simulink model "AcasXuClosedLoop_6"  (R2019b)
settings: Solver=VariableStepAuto  StartTime=0.0  StopTime=30  RelTol=1e-3
libraries: neural x624, simulink x2
(part 1 of 33)
settings Model: Creator=manzand  LastModifiedBy=manzand

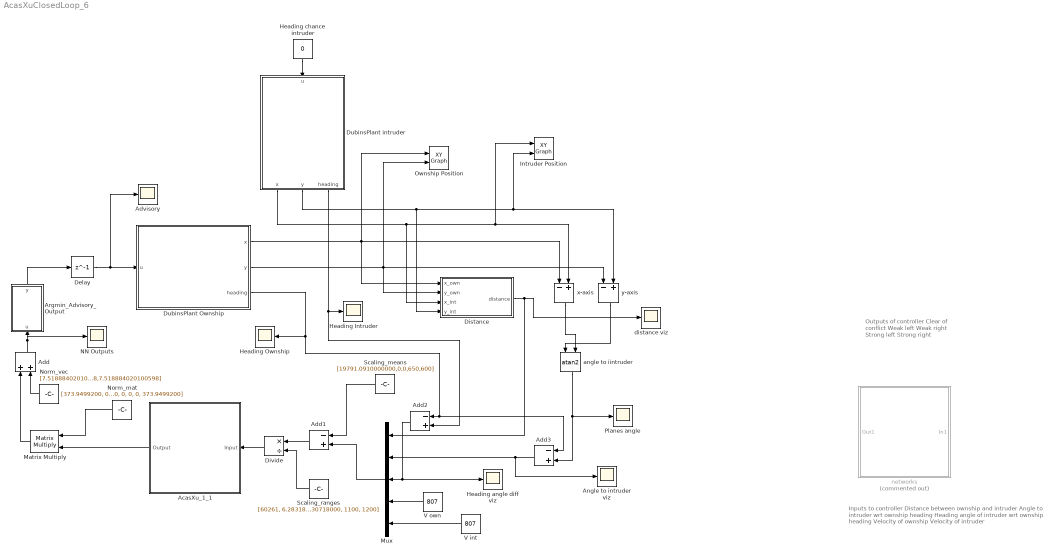
== system AcasXuClosedLoop_6 ==
  note: Outputs of controller
      | Clear of conflict
      | Weak left
      | Weak right
      | Strong left
      | Strong right
  note: Inputs to controller
      | Distance between ownship and intruder
      | Angle to intruder wrt ownship heading
      | Heading angle of intruder wrt ownship heading
      | Velocity of ownship
      | Velocity of intruder
  AcasXu_1_1 : Subsystem
      mask help: Feed-Forward Neural Network
      mask Display: e = 0.06;c1 = [120 150 230]/255;c2 = ([120 150 230]+0)/383;c3 = ([120 150 230]+128)/383;patch([0 1 1 0],[0 0 1 1],c1);patch([0 1 1 1-e 1-e 0+e],[0 0 1 1-e 0+e 0+e],c2);patch([0 0 1 1-e 0+e 0+e],[0 1 1 1-e 1-e 0+e],c3);plot([0 1 1 0 0],[0 0 1 1 0]);fprintf('NNET');port_label('input',1,' Input');port_label('output',1,'Output ');
  Add : Sum  Priority=20
  Add1 : Sum  Priority=14  Inputs=-+
  Add2 : Sum  Priority=9  Inputs=-+
  Add3 : Sum  Priority=9  Inputs=-+
  Advisory : Scope
  Angle to intruder viz : Scope
  Argmin_Advisory_Output : MATLAB Function  Priority=21  TreatAsAtomicUnit=on
  Delay : Delay  Priority=1  DelayLength=1  InitialCondition=0
  Distance : MATLAB Function  Priority=5  TreatAsAtomicUnit=on
  Divide : Product  Priority=16  Inputs=*/
  DubinsPlant Ownship : Stateflow chart  Priority=2  BlockKeywords=__PRM__SERIALIZED__DATA__:Stateflow Chart,Stateflow Diagram  TreatAsAtomicUnit=on
  DubinsPlant intruder : Stateflow chart  Priority=4  BlockKeywords=__PRM__SERIALIZED__DATA__:Stateflow Chart,Stateflow Diagram  TreatAsAtomicUnit=on
  Heading Intruder : Scope
  Heading Ownship : Scope
  Heading angle diff viz : Scope
  "Heading chance intruder " : Constant  Priority=3  Value=0
  Intruder Position : simulink/Sinks/XY Graph  xmin=0  xmax=40200  ymin=-100  ymax=100  st=-1
  Matrix Multiply : Product  Priority=19  Multiplication=Matrix(*)
  Mux : Mux  Priority=12  Inputs=5
  NN Outputs : Scope
  Norm_mat : Constant  Priority=18  Value=|  VectorParams1D=off
      | [373.9499200, 0, 0, 0, 0; 0, 373.9499200, 0, 0, 0;
      | 0, 0, 373.9499200, 0, 0;
      | 0, 0, 0, 373.9499200, 0;
      | 0, 0, 0, 0, 373.9499200]
  "Norm_vec " : Constant  Value=[7.518884020100598, 7.518884020100598,7.518884020100598,7.518884020100598,7.518884020100598]
  Ownship Position : simulink/Sinks/XY Graph  xmin=-500  xmax=8000  ymin=-100  ymax=25000  st=-1
  Planes angle : Scope
  Scaling_means : Constant  Priority=13  Value=[19791.0910000000,0,0,650,600]
  Scaling_ranges : Constant  Priority=15  Value=[60261, 6.28318530718000, 6.28318530718000, 1100, 1200]  VectorParams1D=off
  V int : Constant  Priority=11  Value=807
  V own : Constant  Priority=10  Value=807
  angle to iintruder : Trigonometry  Priority=8  Operator=atan2  OutputSignalType=real
  distance viz : Scope
  networks : Subsystem  Commented=on
  x-axis : Sum  Priority=6  Inputs=-+
  y-axis : Sum  Priority=7  Inputs=-+
  wires:
  Add2/1 -> Mux/3, Heading angle diff viz/1
  V int/1 -> Mux/5
  Mux/1 -> Add1/2
  Argmin_Advisory_Output/1(y) -> Delay/1
  angle to iintruder/1 -> Planes angle/1, Add3/2
  Distance/1(distance) -> Mux/1, distance viz/1
  Scaling_ranges/1 -> Divide/2
  Add1/1 -> Divide/1
  Matrix Multiply/1 -> Add/1
  DubinsPlant intruder/3(heading) -> Heading Intruder/1, Add2/2
  DubinsPlant Ownship/1(x) -> Distance/1(x_own), x-axis/1, Ownship Position/1
  Scaling_means/1 -> Add1/1
  DubinsPlant intruder/2(y) -> Distance/4(y_int), y-axis/2, Intruder Position/2
  "Norm_vec "/1 -> Add/2
  DubinsPlant intruder/1(x) -> Distance/3(x_int), x-axis/2, Intruder Position/1
  Delay/1 -> DubinsPlant Ownship/1(u), Advisory/1
  DubinsPlant Ownship/3(heading) -> Heading Ownship/1, Add3/1, Add2/1
  V own/1 -> Mux/4
  AcasXu_1_1/1(Output) -> Matrix Multiply/2
  "Heading chance intruder "/1 -> DubinsPlant intruder/1(u)
  DubinsPlant Ownship/2(y) -> Distance/2(y_own), y-axis/1, Ownship Position/2
  Add/1 -> NN Outputs/1, Argmin_Advisory_Output/1(u)
  Norm_mat/1 -> Matrix Multiply/1
  Divide/1 -> AcasXu_1_1/1(Input)
  Add3/1 -> Angle to intruder viz/1, Mux/2
  x-axis/1 -> angle to iintruder/2
  y-axis/1 -> angle to iintruder/1

== system AcasXuClosedLoop_6/AcasXu_1_1 ==
  Input : Inport  PortDimensions=5
      mask Display: e = 0.06;c1 = [120 230 180]/255;c2 = ([120 230 180]+0)/(256+128);c3 = ([120 230 180]+128)/(256+128);patch([0 1 1 0],[0 0 1 1],c1);patch([0 1 1 1-e 1-e 0+e],[0 0 1 1-e 0+e 0+e],c2);patch([0 0 1 1-e 0+e 0+e],[0 1 1 1-e 1-e 0+e],c3);plot([0 1 1 0 0],[0 0 1 1 0]);
  Layer 1 : Subsystem
      mask Display: e = 0.06;c1 = [120 150 230]/255;c2 = ([120 150 230]+0)/383;c3 = ([120 150 230]+128)/383;patch([0 1 1 0],[0 0 1 1],c1);patch([0 1 1 1-e 1-e 0+e],[0 0 1 1-e 0+e 0+e],c2);patch([0 0 1 1-e 0+e 0+e],[0 1 1 1-e 1-e 0+e],c3);plot([0 1 1 0 0],[0 0 1 1 0]);
  Layer 2 : Subsystem
      mask Display: e = 0.06;c1 = [120 150 230]/255;c2 = ([120 150 230]+0)/383;c3 = ([120 150 230]+128)/383;patch([0 1 1 0],[0 0 1 1],c1);patch([0 1 1 1-e 1-e 0+e],[0 0 1 1-e 0+e 0+e],c2);patch([0 0 1 1-e 0+e 0+e],[0 1 1 1-e 1-e 0+e],c3);plot([0 1 1 0 0],[0 0 1 1 0]);
  Layer 3 : Subsystem
      mask Display: e = 0.06;c1 = [120 150 230]/255;c2 = ([120 150 230]+0)/383;c3 = ([120 150 230]+128)/383;patch([0 1 1 0],[0 0 1 1],c1);patch([0 1 1 1-e 1-e 0+e],[0 0 1 1-e 0+e 0+e],c2);patch([0 0 1 1-e 0+e 0+e],[0 1 1 1-e 1-e 0+e],c3);plot([0 1 1 0 0],[0 0 1 1 0]);
  Layer 4 : Subsystem
      mask Display: e = 0.06;c1 = [120 150 230]/255;c2 = ([120 150 230]+0)/383;c3 = ([120 150 230]+128)/383;patch([0 1 1 0],[0 0 1 1],c1);patch([0 1 1 1-e 1-e 0+e],[0 0 1 1-e 0+e 0+e],c2);patch([0 0 1 1-e 0+e 0+e],[0 1 1 1-e 1-e 0+e],c3);plot([0 1 1 0 0],[0 0 1 1 0]);
  Layer 5 : Subsystem
      mask Display: e = 0.06;c1 = [120 150 230]/255;c2 = ([120 150 230]+0)/383;c3 = ([120 150 230]+128)/383;patch([0 1 1 0],[0 0 1 1],c1);patch([0 1 1 1-e 1-e 0+e],[0 0 1 1-e 0+e 0+e],c2);patch([0 0 1 1-e 0+e 0+e],[0 1 1 1-e 1-e 0+e],c3);plot([0 1 1 0 0],[0 0 1 1 0]);
  Layer 6 : Subsystem
      mask Display: e = 0.06;c1 = [120 150 230]/255;c2 = ([120 150 230]+0)/383;c3 = ([120 150 230]+128)/383;patch([0 1 1 0],[0 0 1 1],c1);patch([0 1 1 1-e 1-e 0+e],[0 0 1 1-e 0+e 0+e],c2);patch([0 0 1 1-e 0+e 0+e],[0 1 1 1-e 1-e 0+e],c3);plot([0 1 1 0 0],[0 0 1 1 0]);
  Layer 7 : Subsystem
      mask Display: e = 0.06;c1 = [120 150 230]/255;c2 = ([120 150 230]+0)/383;c3 = ([120 150 230]+128)/383;patch([0 1 1 0],[0 0 1 1],c1);patch([0 1 1 1-e 1-e 0+e],[0 0 1 1-e 0+e 0+e],c2);patch([0 0 1 1-e 0+e 0+e],[0 1 1 1-e 1-e 0+e],c3);plot([0 1 1 0 0],[0 0 1 1 0]);
  Process Input 1 : Subsystem
      mask Display: e = 0.06;c1 = [120 150 230]/255;c2 = ([120 150 230]+0)/383;c3 = ([120 150 230]+128)/383;patch([0 1 1 0],[0 0 1 1],c1);patch([0 1 1 1-e 1-e 0+e],[0 0 1 1-e 0+e 0+e],c2);patch([0 0 1 1-e 0+e 0+e],[0 1 1 1-e 1-e 0+e],c3);plot([0 1 1 0 0],[0 0 1 1 0]);
  Process Output 1 : Subsystem
      mask Display: e = 0.06;c1 = [120 150 230]/255;c2 = ([120 150 230]+0)/383;c3 = ([120 150 230]+128)/383;patch([0 1 1 0],[0 0 1 1],c1);patch([0 1 1 1-e 1-e 0+e],[0 0 1 1-e 0+e 0+e],c2);patch([0 0 1 1-e 0+e 0+e],[0 1 1 1-e 1-e 0+e],c3);plot([0 1 1 0 0],[0 0 1 1 0]);
  Output : Outport  InitialOutput=[0;0;0;0;0]
      mask Display: e = 0.06;c1 = [120 230 180]/255;c2 = ([120 230 180]+0)/(256+128);c3 = ([120 230 180]+128)/(256+128);patch([0 1 1 0],[0 0 1 1],c1);patch([0 1 1 1-e 1-e 0+e],[0 0 1 1-e 0+e 0+e],c2);patch([0 0 1 1-e 0+e 0+e],[0 1 1 1-e 1-e 0+e],c3);plot([0 1 1 0 0],[0 0 1 1 0]);
  wires:
  Layer 7/1("a{7}") -> Process Output 1/1(a)
  [feedback6] -> Layer 7/1("a{6} ")
  Layer 6/1("a{6}") -> [feedback6]
  [feedback5] -> Layer 6/1("a{5} ")
  Layer 5/1("a{5}") -> [feedback5]
  [feedback4] -> Layer 5/1("a{4} ")
  Layer 4/1("a{4}") -> [feedback4]
  [feedback3] -> Layer 4/1("a{3} ")
  Layer 3/1("a{3}") -> [feedback3]
  [feedback2] -> Layer 3/1("a{2} ")
  Layer 2/1("a{2}") -> [feedback2]
  [feedback1] -> Layer 2/1("a{1} ")
  Layer 1/1("a{1}") -> [feedback1]
  Process Input 1/1(p) -> Layer 1/1("p{1}")
  Process Output 1/1(y) -> Output/1
  Input/1 -> Process Input 1/1(x)

== system AcasXuClosedLoop_6/networks ==
  In1 : Inport
  AcasXu_5_4 : Subsystem  Priority=17
      mask help: Feed-Forward Neural Network
      mask Display: e = 0.06;c1 = [120 150 230]/255;c2 = ([120 150 230]+0)/383;c3 = ([120 150 230]+128)/383;patch([0 1 1 0],[0 0 1 1],c1);patch([0 1 1 1-e 1-e 0+e],[0 0 1 1-e 0+e 0+e],c2);patch([0 0 1 1-e 0+e 0+e],[0 1 1 1-e 1-e 0+e],c3);plot([0 1 1 0 0],[0 0 1 1 0]);fprintf('NNET');port_label('input',1,' Input');port_label('output',1,'Output ');
  Out1 : Outport
  wires:
  In1/1 -> AcasXu_5_4/1(Input)
  AcasXu_5_4/1(Output) -> Out1/1

== system AcasXuClosedLoop_6/AcasXu_1_1/Layer 1 ==
  "p{1}" : Inport  PortDimensions=5
      mask Display: e = 0.06;c1 = [120 230 180]/255;c2 = ([120 230 180]+0)/(256+128);c3 = ([120 230 180]+128)/(256+128);patch([0 1 1 0],[0 0 1 1],c1);patch([0 1 1 1-e 1-e 0+e],[0 0 1 1-e 0+e 0+e],c2);patch([0 0 1 1-e 0+e 0+e],[0 1 1 1-e 1-e 0+e],c3);plot([0 1 1 0 0],[0 0 1 1 0]);
  Delays 1 : Subsystem
      mask Display: e = 0.06;c1 = [120 150 230]/255;c2 = ([120 150 230]+0)/383;c3 = ([120 150 230]+128)/383;patch([0 1 1 0],[0 0 1 1],c1);patch([0 1 1 1-e 1-e 0+e],[0 0 1 1-e 0+e 0+e],c2);patch([0 0 1 1-e 0+e 0+e],[0 1 1 1-e 1-e 0+e],c3);plot([0 1 1 0 0],[0 0 1 1 0]);disp('0');
  "IW{1,1}" : Subsystem
      mask Display: e = 0.06;c1 = [120 150 230]/255;c2 = ([120 150 230]+0)/383;c3 = ([120 150 230]+128)/383;patch([0 1 1 0],[0 0 1 1],c1);patch([0 1 1 1-e 1-e 0+e],[0 0 1 1-e 0+e 0+e],c2);patch([0 0 1 1-e 0+e 0+e],[0 1 1 1-e 1-e 0+e],c3);plot([0 1 1 0 0],[0 0 1 1 0]);disp('W');
  "b{1}" : Constant  Value=[0.227629999999999999005240169935859739780426025390625;-0.1887620000000000131112898316132486797869205474853515625;0.053409400000000002706190826984311570413410663604736328125;-0.3778610000000000024300561562995426356792449951171875;-0.0812530999999999947736029071165830828249454498291015625;-0.588651000000000035328184821992181241512298583984375;0.07460650000000000614530648590516648255288600921630859375;-0.3928869999999999862438926356844604015350341796875;-0.356302999999999980840215130228898487985134124755859375;-0.1677119999999999999662492200513952411711215972900390625;0.058710900000000003362554679142704117111861705780029296875;0.18391699999999999715072362960199825465679168701171875;0.13195699999999999096900182848912663757801055908203125;-0.30868099999999998317434801720082759857177734375;0.1969289999999999929425342770628049038350582122802734375;0.2066639999999999866009403604039107449352741241455078125;-0.311695999999999973084641169407404959201812744140625;0.030657600000000000128874688698488171212375164031982421875;-0.1388220000000000009521272659185342490673065185546875;-0.3474340000000000205915284823277033865451812744140625;-0.004518399999999999673561124069465222419239580631256103515625;-0.390616000000000018754775510387844406068325042724609375;0.09696349999999999413891060839887359179556369781494140625;0.009832660000000000011244338793403585441410541534423828125;-0.01885850000000000026290081223123706877231597900390625;-0.231918999999999986272314345114864408969879150390625;-0.2381649999999999878230738659112830646336078643798828125;0.07101480000000000292192936512947198934853076934814453125;-0.141913000000000011358025631125201471149921417236328125;-0.442307000000000005712763595511205494403839111328125;0.55908400000000002538769194870837964117527008056640625;0.1354829999999999923243620969515177421271800994873046875;-0.37321700000000002095390527756535448133945465087890625;-0.415389999999999981472598165055387653410434722900390625;0.7596380000000000354276608049985952675342559814453125;0.1328249999999999986233234494648058898746967315673828125;0.235565999999999997616129121524863876402378082275390625;0.214857999999999993434585121576674282550811767578125;-0.440840999999999982872367354502785019576549530029296875;-0.077296799999999998842525883446796797215938568115234375;0.2216059999999999974296116533878375776112079620361328125;-0.006508729999999999897564162409935306641273200511932373046875;-0.634843000000000046156856114976108074188232421875;-0.15383299999999999752020585219725035130977630615234375;-0.05730269999999999808171224913166952319443225860595703125;-0.10922900000000000664268640093723661266267299652099609375;0.037034400000000002040057012209217646159231662750244140625;0.05380870000000000097362118367527727968990802764892578125;-0.44755000000000000337507799486047588288784027099609375;0.17591699999999999004529627200099639594554901123046875]
      mask Display: e = 0.06;c1 = [120 150 230]/255;c2 = ([120 150 230]+0)/383;c3 = ([120 150 230]+128)/383;patch([0 1 1 0],[0 0 1 1],c1);patch([0 1 1 1-e 1-e 0+e],[0 0 1 1-e 0+e 0+e],c2);patch([0 0 1 1-e 0+e 0+e],[0 1 1 1-e 1-e 0+e],c3);plot([0 1 1 0 0],[0 0 1 1 0]);disp('b');
  netsum : Sum  Inputs=2  SaturateOnIntegerOverflow=on  InputSameDT=on  OutDataTypeStr=Inherit: Same as first input
      mask Display: e = 0.06;c1 = [120 150 230]/255;c2 = ([120 150 230]+0)/383;c3 = ([120 150 230]+128)/383;patch([0 1 1 0],[0 0 1 1],c1);patch([0 1 1 1-e 1-e 0+e],[0 0 1 1-e 0+e 0+e],c2);patch([0 0 1 1-e 0+e 0+e],[0 1 1 1-e 1-e 0+e],c3);plot([0 1 1 0 0],[0 0 1 1 0]);disp('+');
  tansig : neural/Transfer Functions/tansig
      settings: SourceProductName=Deep Learning Toolbox
  "a{1}" : Outport  InitialOutput=[0;0;0;0;0;0;0;0;0;0;0;0;0;0;0;0;0;0;0;0;0;0;0;0;0;0;0;0;0;0;0;0;0;0;0;0;0;0;0;0;0;0;0;0;0;0;0;0;0;0]
      mask Display: e = 0.06;c1 = [120 230 180]/255;c2 = ([120 230 180]+0)/(256+128);c3 = ([120 230 180]+128)/(256+128);patch([0 1 1 0],[0 0 1 1],c1);patch([0 1 1 1-e 1-e 0+e],[0 0 1 1-e 0+e 0+e],c2);patch([0 0 1 1-e 0+e 0+e],[0 1 1 1-e 1-e 0+e],c3);plot([0 1 1 0 0],[0 0 1 1 0]);
  wires:
  tansig/1 -> "a{1}"/1
  netsum/1 -> tansig/1
  "b{1}"/1 -> netsum/2
  "IW{1,1}"/1("iz{1,1}") -> netsum/1
  Delays 1/1("pd{1,1}") -> "IW{1,1}"/1("pd{1,1}")
  "p{1}"/1 -> Delays 1/1("p{1}")

== system AcasXuClosedLoop_6/AcasXu_1_1/Layer 2 ==
  "a{1} " : Inport  PortDimensions=50
      mask Display: e = 0.06;c1 = [120 230 180]/255;c2 = ([120 230 180]+0)/(256+128);c3 = ([120 230 180]+128)/(256+128);patch([0 1 1 0],[0 0 1 1],c1);patch([0 1 1 1-e 1-e 0+e],[0 0 1 1-e 0+e 0+e],c2);patch([0 0 1 1-e 0+e 0+e],[0 1 1 1-e 1-e 0+e],c3);plot([0 1 1 0 0],[0 0 1 1 0]);
  Delays 1 : Subsystem
      mask Display: e = 0.06;c1 = [120 150 230]/255;c2 = ([120 150 230]+0)/383;c3 = ([120 150 230]+128)/383;patch([0 1 1 0],[0 0 1 1],c1);patch([0 1 1 1-e 1-e 0+e],[0 0 1 1-e 0+e 0+e],c2);patch([0 0 1 1-e 0+e 0+e],[0 1 1 1-e 1-e 0+e],c3);plot([0 1 1 0 0],[0 0 1 1 0]);disp('0');
  "LW{2,1}" : Subsystem
      mask Display: e = 0.06;c1 = [120 150 230]/255;c2 = ([120 150 230]+0)/383;c3 = ([120 150 230]+128)/383;patch([0 1 1 0],[0 0 1 1],c1);patch([0 1 1 1-e 1-e 0+e],[0 0 1 1-e 0+e 0+e],c2);patch([0 0 1 1-e 0+e 0+e],[0 1 1 1-e 1-e 0+e],c3);plot([0 1 1 0 0],[0 0 1 1 0]);disp('W');
  "b{2}" : Constant  Value=[0.08354999999999999926725280374739668332040309906005859375;-0.02132610000000000061159965980550623498857021331787109375;0.75629100000000004655476004700176417827606201171875;-1.25082000000000004291678123991005122661590576171875;0.1784689999999999887592139202752150595188140869140625;-0.339158000000000015017320720289717428386211395263671875;0.10922600000000000364241969919021357782185077667236328125;-1.262140000000000039648284655413590371608734130859375;-0.35648800000000002707878365981741808354854583740234375;-0.00829379000000000053682835954305119230411946773529052734375;-0.020118299999999998683986035530324443243443965911865234375;-0.1920389999999999874891187801040359772741794586181640625;-0.089257799999999998252775412765913642942905426025390625;-0.2063190000000000023927526626721373759210109710693359375;0.10505299999999999360777991341819870285689830780029296875;-0.09322260000000000268460809138559852726757526397705078125;-0.2459240000000000037072567238283227197825908660888671875;0.1594160000000000021458390619955025613307952880859375;0.465793999999999985828225135264801792800426483154296875;-0.76003900000000002012967570408363826572895050048828125;0.1272129999999999927506877384075778536498546600341796875;0.393189000000000010714984455262310802936553955078125;-0.071787199999999995458921375757199712097644805908203125;0.3198309999999999764241920274798758327960968017578125;-0.0141183000000000002938094212368014268577098846435546875;-0.00660377000000000012602807686334926984272897243499755859375;-0.7037139999999999506741232835338450968265533447265625;0.44089400000000000812150346973794512450695037841796875;-0.403874000000000010768275160444318316876888275146484375;-0.55025800000000002487610117896110750734806060791015625;-1.3335500000000000131450406115618534386157989501953125;-1.1195600000000001106315039578475989401340484619140625;-0.7316730000000000178062009581481106579303741455078125;0.237414999999999987156940051136189140379428863525390625;-0.8274880000000000013216094885137863457202911376953125;0.317529000000000005687894599759601987898349761962890625;-0.74180100000000004367706196717335842549800872802734375;-0.0174412000000000004529265851260788622312247753143310546875;-0.3022059999999999746478351880796253681182861328125;-0.099699399999999993582378010614775121212005615234375;0.6550789999999999668744976588641293346881866455078125;1.2524100000000000232347474593552760779857635498046875;0.03909870000000000012096990076315705664455890655517578125;-0.02423820000000000141060496616773889400064945220947265625;-0.385695999999999983298692995958845131099224090576171875;-0.359070999999999973528730379257467575371265411376953125;-0.155855999999999994543031789362430572509765625;0.02859710000000000029718449923166190274059772491455078125;-0.4266229999999999744630940767819993197917938232421875;0.78092499999999998028243908265721984207630157470703125]
      mask Display: e = 0.06;c1 = [120 150 230]/255;c2 = ([120 150 230]+0)/383;c3 = ([120 150 230]+128)/383;patch([0 1 1 0],[0 0 1 1],c1);patch([0 1 1 1-e 1-e 0+e],[0 0 1 1-e 0+e 0+e],c2);patch([0 0 1 1-e 0+e 0+e],[0 1 1 1-e 1-e 0+e],c3);plot([0 1 1 0 0],[0 0 1 1 0]);disp('b');
  netsum : Sum  Inputs=2  SaturateOnIntegerOverflow=on  InputSameDT=on  OutDataTypeStr=Inherit: Same as first input
      mask Display: e = 0.06;c1 = [120 150 230]/255;c2 = ([120 150 230]+0)/383;c3 = ([120 150 230]+128)/383;patch([0 1 1 0],[0 0 1 1],c1);patch([0 1 1 1-e 1-e 0+e],[0 0 1 1-e 0+e 0+e],c2);patch([0 0 1 1-e 0+e 0+e],[0 1 1 1-e 1-e 0+e],c3);plot([0 1 1 0 0],[0 0 1 1 0]);disp('+');
  tansig : neural/Transfer Functions/tansig
      settings: SourceProductName=Deep Learning Toolbox
  "a{2}" : Outport  InitialOutput=[0;0;0;0;0;0;0;0;0;0;0;0;0;0;0;0;0;0;0;0;0;0;0;0;0;0;0;0;0;0;0;0;0;0;0;0;0;0;0;0;0;0;0;0;0;0;0;0;0;0]
      mask Display: e = 0.06;c1 = [120 230 180]/255;c2 = ([120 230 180]+0)/(256+128);c3 = ([120 230 180]+128)/(256+128);patch([0 1 1 0],[0 0 1 1],c1);patch([0 1 1 1-e 1-e 0+e],[0 0 1 1-e 0+e 0+e],c2);patch([0 0 1 1-e 0+e 0+e],[0 1 1 1-e 1-e 0+e],c3);plot([0 1 1 0 0],[0 0 1 1 0]);
  wires:
  tansig/1 -> "a{2}"/1
  netsum/1 -> tansig/1
  "b{2}"/1 -> netsum/2
  "LW{2,1}"/1("lz{2,1}") -> netsum/1
  Delays 1/1("pd{2,1}") -> "LW{2,1}"/1("ad{2,1}")
  "a{1} "/1 -> Delays 1/1("p{2}")

== system AcasXuClosedLoop_6/AcasXu_1_1/Layer 3 ==
  "a{2} " : Inport  PortDimensions=50
      mask Display: e = 0.06;c1 = [120 230 180]/255;c2 = ([120 230 180]+0)/(256+128);c3 = ([120 230 180]+128)/(256+128);patch([0 1 1 0],[0 0 1 1],c1);patch([0 1 1 1-e 1-e 0+e],[0 0 1 1-e 0+e 0+e],c2);patch([0 0 1 1-e 0+e 0+e],[0 1 1 1-e 1-e 0+e],c3);plot([0 1 1 0 0],[0 0 1 1 0]);
  Delays 1 : Subsystem
      mask Display: e = 0.06;c1 = [120 150 230]/255;c2 = ([120 150 230]+0)/383;c3 = ([120 150 230]+128)/383;patch([0 1 1 0],[0 0 1 1],c1);patch([0 1 1 1-e 1-e 0+e],[0 0 1 1-e 0+e 0+e],c2);patch([0 0 1 1-e 0+e 0+e],[0 1 1 1-e 1-e 0+e],c3);plot([0 1 1 0 0],[0 0 1 1 0]);disp('0');
  "LW{3,2}" : Subsystem
      mask Display: e = 0.06;c1 = [120 150 230]/255;c2 = ([120 150 230]+0)/383;c3 = ([120 150 230]+128)/383;patch([0 1 1 0],[0 0 1 1],c1);patch([0 1 1 1-e 1-e 0+e],[0 0 1 1-e 0+e 0+e],c2);patch([0 0 1 1-e 0+e 0+e],[0 1 1 1-e 1-e 0+e],c3);plot([0 1 1 0 0],[0 0 1 1 0]);disp('W');
  "b{3}" : Constant  Value=[-0.40848600000000001575273245180142112076282501220703125;1.068750000000000088817841970012523233890533447265625;-0.1013509999999999966480146440517273731529712677001953125;0.291739000000000026080471116074477322399616241455078125;0.361906000000000005467626351673970930278301239013671875;-1.17598000000000002529532139305956661701202392578125;-1.084940000000000015489831639570184051990509033203125;-0.5253959999999999741504552730475552380084991455078125;-0.48512100000000002442135382807464338839054107666015625;-0.56345100000000003515054913805215619504451751708984375;-0.430958000000000007734257678748690523207187652587890625;-0.375101999999999990986765396883129142224788665771484375;-0.299368999999999996219912645756267011165618896484375;-0.300263000000000002120970066243899054825305938720703125;-0.52805800000000002736300075412145815789699554443359375;-0.062003200000000001368416491231982945464551448822021484375;-0.65378999999999998227195874278550036251544952392578125;0.7301809999999999689634933019988238811492919921875;-0.849960999999999966547648000414483249187469482421875;-0.0157297999999999986442400512487438390962779521942138671875;-0.289808000000000010043521569969016127288341522216796875;0.278940000000000021262991367620998062193393707275390625;1.470779999999999976267872625612653791904449462890625;2.107930000000000081428197518107481300830841064453125;-0.310170000000000001261213355974177829921245574951171875;-0.53844400000000003370104195710155181586742401123046875;-0.1459189999999999931556970977908349595963954925537109375;1.0104900000000001103472868635435588657855987548828125;-0.374155999999999988592236377371591515839099884033203125;-0.052722199999999996844479710489395074546337127685546875;-0.1487900000000000055866422599137877114117145538330078125;0.25546400000000002439293211864423938095569610595703125;-0.77219800000000005102407385493279434740543365478515625;-1.7604699999999999793232063893810845911502838134765625;0.062296600000000000585398396424352540634572505950927734375;0.254439000000000026258106800014502368867397308349609375;-0.150743999999999989114485288155265152454376220703125;-0.75726400000000004819611376660759560763835906982421875;-2.46424999999999982946974341757595539093017578125;-0.91319399999999995021227050528977997601032257080078125;-0.56305799999999994742694298111018724739551544189453125;-0.217100999999999988432364261825568974018096923828125;0.5705459999999999975983655531308613717555999755859375;-0.52340799999999998437516524063539691269397735595703125;-1.4999700000000000255084842137875966727733612060546875;-0.261921000000000014917844737283303402364253997802734375;-0.52610900000000004883560222879168577492237091064453125;-0.0059898399999999997478372648629374452866613864898681640625;-0.464336000000000026499691330172936432063579559326171875;0.11419500000000000483613149526718189008533954620361328125]
      mask Display: e = 0.06;c1 = [120 150 230]/255;c2 = ([120 150 230]+0)/383;c3 = ([120 150 230]+128)/383;patch([0 1 1 0],[0 0 1 1],c1);patch([0 1 1 1-e 1-e 0+e],[0 0 1 1-e 0+e 0+e],c2);patch([0 0 1 1-e 0+e 0+e],[0 1 1 1-e 1-e 0+e],c3);plot([0 1 1 0 0],[0 0 1 1 0]);disp('b');
  netsum : Sum  Inputs=2  SaturateOnIntegerOverflow=on  InputSameDT=on  OutDataTypeStr=Inherit: Same as first input
      mask Display: e = 0.06;c1 = [120 150 230]/255;c2 = ([120 150 230]+0)/383;c3 = ([120 150 230]+128)/383;patch([0 1 1 0],[0 0 1 1],c1);patch([0 1 1 1-e 1-e 0+e],[0 0 1 1-e 0+e 0+e],c2);patch([0 0 1 1-e 0+e 0+e],[0 1 1 1-e 1-e 0+e],c3);plot([0 1 1 0 0],[0 0 1 1 0]);disp('+');
  tansig : neural/Transfer Functions/tansig
      settings: SourceProductName=Deep Learning Toolbox
  "a{3}" : Outport  InitialOutput=[0;0;0;0;0;0;0;0;0;0;0;0;0;0;0;0;0;0;0;0;0;0;0;0;0;0;0;0;0;0;0;0;0;0;0;0;0;0;0;0;0;0;0;0;0;0;0;0;0;0]
      mask Display: e = 0.06;c1 = [120 230 180]/255;c2 = ([120 230 180]+0)/(256+128);c3 = ([120 230 180]+128)/(256+128);patch([0 1 1 0],[0 0 1 1],c1);patch([0 1 1 1-e 1-e 0+e],[0 0 1 1-e 0+e 0+e],c2);patch([0 0 1 1-e 0+e 0+e],[0 1 1 1-e 1-e 0+e],c3);plot([0 1 1 0 0],[0 0 1 1 0]);
  wires:
  tansig/1 -> "a{3}"/1
  netsum/1 -> tansig/1
  "b{3}"/1 -> netsum/2
  "LW{3,2}"/1("lz{3,2}") -> netsum/1
  Delays 1/1("pd{3,2}") -> "LW{3,2}"/1("ad{3,2}")
  "a{2} "/1 -> Delays 1/1("p{3}")

== system AcasXuClosedLoop_6/AcasXu_1_1/Layer 4 ==
  "a{3} " : Inport  PortDimensions=50
      mask Display: e = 0.06;c1 = [120 230 180]/255;c2 = ([120 230 180]+0)/(256+128);c3 = ([120 230 180]+128)/(256+128);patch([0 1 1 0],[0 0 1 1],c1);patch([0 1 1 1-e 1-e 0+e],[0 0 1 1-e 0+e 0+e],c2);patch([0 0 1 1-e 0+e 0+e],[0 1 1 1-e 1-e 0+e],c3);plot([0 1 1 0 0],[0 0 1 1 0]);
  Delays 1 : Subsystem
      mask Display: e = 0.06;c1 = [120 150 230]/255;c2 = ([120 150 230]+0)/383;c3 = ([120 150 230]+128)/383;patch([0 1 1 0],[0 0 1 1],c1);patch([0 1 1 1-e 1-e 0+e],[0 0 1 1-e 0+e 0+e],c2);patch([0 0 1 1-e 0+e 0+e],[0 1 1 1-e 1-e 0+e],c3);plot([0 1 1 0 0],[0 0 1 1 0]);disp('0');
  "LW{4,3}" : Subsystem
      mask Display: e = 0.06;c1 = [120 150 230]/255;c2 = ([120 150 230]+0)/383;c3 = ([120 150 230]+128)/383;patch([0 1 1 0],[0 0 1 1],c1);patch([0 1 1 1-e 1-e 0+e],[0 0 1 1-e 0+e 0+e],c2);patch([0 0 1 1-e 0+e 0+e],[0 1 1 1-e 1-e 0+e],c3);plot([0 1 1 0 0],[0 0 1 1 0]);disp('W');
  "b{4}" : Constant  Value=[1.4841599999999999237587644529412500560283660888671875;-0.039272700000000000664091004409783636219799518585205078125;-0.0907837999999999978317788418280542828142642974853515625;-2.473970000000000002415845301584340631961822509765625;-2.268639999999999989910293152206577360630035400390625;0.289910999999999974274800251805572770535945892333984375;0.08497839999999999560653662911136052571237087249755859375;-0.0216935000000000009767742170652127242647111415863037109375;-0.68817300000000003468159093245049007236957550048828125;-0.2453579999999999927684513068015803582966327667236328125;-0.40888299999999999645439174855710007250308990478515625;0.345316000000000011826983836726867593824863433837890625;-1.175380000000000091375795818748883903026580810546875;-0.129693000000000002724931391639984212815761566162109375;-0.01538130000000000052740034561793436296284198760986328125;2.3029799999999998050270733074285089969635009765625;0.472198999999999979859666154879960231482982635498046875;-0.466608999999999995988986256634234450757503509521484375;-1.123510000000000008668621376273222267627716064453125;0.495937000000000016708412431398755870759487152099609375;-0.570643000000000011340262062731198966503143310546875;-0.78851499999999996592947582030319608747959136962890625;1.0165200000000000901678731679567135870456695556640625;0.462602000000000013191225889386259950697422027587890625;-1.629129999999999967030817060731351375579833984375;-0.58421500000000003982592033935361541807651519775390625;0.124253000000000002334132886971929110586643218994140625;-0.077460699999999993448085433556116186082363128662109375;0.288895999999999986140863938999245874583721160888671875;-1.9272199999999999331379285649745725095272064208984375;-1.8612800000000000455457893622224219143390655517578125;0.50749900000000003341682486279751174151897430419921875;2.08643000000000000682121026329696178436279296875;-0.10097499999999999531485883608183939941227436065673828125;0.302989000000000008316902722071972675621509552001953125;-0.80088499999999995804245145336608402431011199951171875;-0.1665010000000000101039177025086246430873870849609375;0.2249150000000000038102854205135372467339038848876953125;-0.31376999999999999335642542064306326210498809814453125;-0.0885139000000000064627414531059912405908107757568359375;-0.041322799999999999809308093290383112616837024688720703125;-0.68847800000000003439737383814644999802112579345703125;0.0999729000000000034287239714103634469211101531982421875;0.2356930000000000136051170329665183089673519134521484375;0.200207999999999997076116642347187735140323638916015625;0.1853219999999999867412725507165305316448211669921875;0.213241999999999987114307486990583129227161407470703125;-0.036336399999999997867394796458029304631054401397705078125;0.07628369999999999595541311236956971697509288787841796875;-0.216393000000000002014388655879884026944637298583984375]
      mask Display: e = 0.06;c1 = [120 150 230]/255;c2 = ([120 150 230]+0)/383;c3 = ([120 150 230]+128)/383;patch([0 1 1 0],[0 0 1 1],c1);patch([0 1 1 1-e 1-e 0+e],[0 0 1 1-e 0+e 0+e],c2);patch([0 0 1 1-e 0+e 0+e],[0 1 1 1-e 1-e 0+e],c3);plot([0 1 1 0 0],[0 0 1 1 0]);disp('b');
  netsum : Sum  Inputs=2  SaturateOnIntegerOverflow=on  InputSameDT=on  OutDataTypeStr=Inherit: Same as first input
      mask Display: e = 0.06;c1 = [120 150 230]/255;c2 = ([120 150 230]+0)/383;c3 = ([120 150 230]+128)/383;patch([0 1 1 0],[0 0 1 1],c1);patch([0 1 1 1-e 1-e 0+e],[0 0 1 1-e 0+e 0+e],c2);patch([0 0 1 1-e 0+e 0+e],[0 1 1 1-e 1-e 0+e],c3);plot([0 1 1 0 0],[0 0 1 1 0]);disp('+');
  tansig : neural/Transfer Functions/tansig
      settings: SourceProductName=Deep Learning Toolbox
  "a{4}" : Outport  InitialOutput=[0;0;0;0;0;0;0;0;0;0;0;0;0;0;0;0;0;0;0;0;0;0;0;0;0;0;0;0;0;0;0;0;0;0;0;0;0;0;0;0;0;0;0;0;0;0;0;0;0;0]
      mask Display: e = 0.06;c1 = [120 230 180]/255;c2 = ([120 230 180]+0)/(256+128);c3 = ([120 230 180]+128)/(256+128);patch([0 1 1 0],[0 0 1 1],c1);patch([0 1 1 1-e 1-e 0+e],[0 0 1 1-e 0+e 0+e],c2);patch([0 0 1 1-e 0+e 0+e],[0 1 1 1-e 1-e 0+e],c3);plot([0 1 1 0 0],[0 0 1 1 0]);
  wires:
  tansig/1 -> "a{4}"/1
  netsum/1 -> tansig/1
  "b{4}"/1 -> netsum/2
  "LW{4,3}"/1("lz{4,3}") -> netsum/1
  Delays 1/1("pd{4,3}") -> "LW{4,3}"/1("ad{4,3}")
  "a{3} "/1 -> Delays 1/1("p{4}")

== system AcasXuClosedLoop_6/AcasXu_1_1/Layer 5 ==
  "a{4} " : Inport  PortDimensions=50
      mask Display: e = 0.06;c1 = [120 230 180]/255;c2 = ([120 230 180]+0)/(256+128);c3 = ([120 230 180]+128)/(256+128);patch([0 1 1 0],[0 0 1 1],c1);patch([0 1 1 1-e 1-e 0+e],[0 0 1 1-e 0+e 0+e],c2);patch([0 0 1 1-e 0+e 0+e],[0 1 1 1-e 1-e 0+e],c3);plot([0 1 1 0 0],[0 0 1 1 0]);
  Delays 1 : Subsystem
      mask Display: e = 0.06;c1 = [120 150 230]/255;c2 = ([120 150 230]+0)/383;c3 = ([120 150 230]+128)/383;patch([0 1 1 0],[0 0 1 1],c1);patch([0 1 1 1-e 1-e 0+e],[0 0 1 1-e 0+e 0+e],c2);patch([0 0 1 1-e 0+e 0+e],[0 1 1 1-e 1-e 0+e],c3);plot([0 1 1 0 0],[0 0 1 1 0]);disp('0');
  "LW{5,4}" : Subsystem
      mask Display: e = 0.06;c1 = [120 150 230]/255;c2 = ([120 150 230]+0)/383;c3 = ([120 150 230]+128)/383;patch([0 1 1 0],[0 0 1 1],c1);patch([0 1 1 1-e 1-e 0+e],[0 0 1 1-e 0+e 0+e],c2);patch([0 0 1 1-e 0+e 0+e],[0 1 1 1-e 1-e 0+e],c3);plot([0 1 1 0 0],[0 0 1 1 0]);disp('W');
  "b{5}" : Constant  Value=[0.343884000000000022989610215518041513860225677490234375;-0.148704000000000002845723656719201244413852691650390625;-0.182344000000000006078693104427657090127468109130859375;2.092820000000000124629195852321572601795196533203125;0.057392100000000001447375552743324078619480133056640625;1.0727800000000000668620714350254274904727935791015625;-3.537500000000000088817841970012523233890533447265625;0.2902460000000000039932501749717630445957183837890625;1.7852799999999999780442294650129042565822601318359375;0.5703920000000000101181285572238266468048095703125;0.102578000000000002511768570911954157054424285888671875;-0.8676939999999999653113036401919089257717132568359375;-1.8884399999999998964739233997534029185771942138671875;-1.11488999999999993661958797019906342029571533203125;-0.445674999999999987831955650108284316956996917724609375;0.694015999999999966263430906110443174839019775390625;1.2776199999999999779021209178608842194080352783203125;-1.2911200000000000454036808150704018771648406982421875;-1.34224999999999994315658113919198513031005859375;-0.15967100000000000736832816983223892748355865478515625;0.64522299999999999098321268320432864129543304443359375;0.988628999999999980019538270425982773303985595703125;0.5161510000000000264464006249909289181232452392578125;-2.3827400000000000801492205937393009662628173828125;0.67675600000000002420819100734661333262920379638671875;0.76186699999999996091304410583688877522945404052734375;0.056760600000000001330580090552757610566914081573486328125;-0.2224609999999999920827775667930836789309978485107421875;1.869569999999999954098939269897527992725372314453125;1.052049999999999929656269159750081598758697509765625;-0.1076290000000000024460433678541448898613452911376953125;0.0906623000000000012210676914037321694195270538330078125;2.556319999999999925677229839493520557880401611328125;0.87517400000000000748201500755385495722293853759765625;0.08279160000000000685371759345798636786639690399169921875;-1.1624499999999999833022457096376456320285797119140625;1.1968300000000000604671868131845258176326751708984375;0.11945899999999999574473719121670001186430454254150390625;0.052382600000000001383426706524915061891078948974609375;-0.25143999999999999683808482586755417287349700927734375;0.9712009999999999809716655363445170223712921142578125;0.41452299999999997481836544466204941272735595703125;0.55931600000000003536371195878018625080585479736328125;0.71126500000000003609557097661308944225311279296875;-3.244779999999999997584154698415659368038177490234375;0.57999999999999996003197111349436454474925994873046875;0.165872999999999992670751680634566582739353179931640625;-1.2932699999999999196376165855326689779758453369140625;-0.331040999999999974168218841441557742655277252197265625;-0.65416499999999999648281345798750407993793487548828125]
      mask Display: e = 0.06;c1 = [120 150 230]/255;c2 = ([120 150 230]+0)/383;c3 = ([120 150 230]+128)/383;patch([0 1 1 0],[0 0 1 1],c1);patch([0 1 1 1-e 1-e 0+e],[0 0 1 1-e 0+e 0+e],c2);patch([0 0 1 1-e 0+e 0+e],[0 1 1 1-e 1-e 0+e],c3);plot([0 1 1 0 0],[0 0 1 1 0]);disp('b');
  netsum : Sum  Inputs=2  SaturateOnIntegerOverflow=on  InputSameDT=on  OutDataTypeStr=Inherit: Same as first input
      mask Display: e = 0.06;c1 = [120 150 230]/255;c2 = ([120 150 230]+0)/383;c3 = ([120 150 230]+128)/383;patch([0 1 1 0],[0 0 1 1],c1);patch([0 1 1 1-e 1-e 0+e],[0 0 1 1-e 0+e 0+e],c2);patch([0 0 1 1-e 0+e 0+e],[0 1 1 1-e 1-e 0+e],c3);plot([0 1 1 0 0],[0 0 1 1 0]);disp('+');
  tansig : neural/Transfer Functions/tansig
      settings: SourceProductName=Deep Learning Toolbox
  "a{5}" : Outport  InitialOutput=[0;0;0;0;0;0;0;0;0;0;0;0;0;0;0;0;0;0;0;0;0;0;0;0;0;0;0;0;0;0;0;0;0;0;0;0;0;0;0;0;0;0;0;0;0;0;0;0;0;0]
      mask Display: e = 0.06;c1 = [120 230 180]/255;c2 = ([120 230 180]+0)/(256+128);c3 = ([120 230 180]+128)/(256+128);patch([0 1 1 0],[0 0 1 1],c1);patch([0 1 1 1-e 1-e 0+e],[0 0 1 1-e 0+e 0+e],c2);patch([0 0 1 1-e 0+e 0+e],[0 1 1 1-e 1-e 0+e],c3);plot([0 1 1 0 0],[0 0 1 1 0]);
  wires:
  tansig/1 -> "a{5}"/1
  netsum/1 -> tansig/1
  "b{5}"/1 -> netsum/2
  "LW{5,4}"/1("lz{5,4}") -> netsum/1
  Delays 1/1("pd{5,4}") -> "LW{5,4}"/1("ad{5,4}")
  "a{4} "/1 -> Delays 1/1("p{5}")

== system AcasXuClosedLoop_6/AcasXu_1_1/Layer 6 ==
  "a{5} " : Inport  PortDimensions=50
      mask Display: e = 0.06;c1 = [120 230 180]/255;c2 = ([120 230 180]+0)/(256+128);c3 = ([120 230 180]+128)/(256+128);patch([0 1 1 0],[0 0 1 1],c1);patch([0 1 1 1-e 1-e 0+e],[0 0 1 1-e 0+e 0+e],c2);patch([0 0 1 1-e 0+e 0+e],[0 1 1 1-e 1-e 0+e],c3);plot([0 1 1 0 0],[0 0 1 1 0]);
  Delays 1 : Subsystem
      mask Display: e = 0.06;c1 = [120 150 230]/255;c2 = ([120 150 230]+0)/383;c3 = ([120 150 230]+128)/383;patch([0 1 1 0],[0 0 1 1],c1);patch([0 1 1 1-e 1-e 0+e],[0 0 1 1-e 0+e 0+e],c2);patch([0 0 1 1-e 0+e 0+e],[0 1 1 1-e 1-e 0+e],c3);plot([0 1 1 0 0],[0 0 1 1 0]);disp('0');
  "LW{6,5}" : Subsystem
      mask Display: e = 0.06;c1 = [120 150 230]/255;c2 = ([120 150 230]+0)/383;c3 = ([120 150 230]+128)/383;patch([0 1 1 0],[0 0 1 1],c1);patch([0 1 1 1-e 1-e 0+e],[0 0 1 1-e 0+e 0+e],c2);patch([0 0 1 1-e 0+e 0+e],[0 1 1 1-e 1-e 0+e],c3);plot([0 1 1 0 0],[0 0 1 1 0]);disp('W');
  "b{6}" : Constant  Value=[-0.4300610000000000265885091721429489552974700927734375;-0.0245742000000000009041212223337424802593886852264404296875;-1.857369999999999965467623042059130966663360595703125;-0.0138151999999999997026378650843980722129344940185546875;0.419246999999999980790477138725691474974155426025390625;-0.2135869999999999990780708003512700088322162628173828125;0.160069999999999990070165267752599902451038360595703125;0.741837999999999997413624441833235323429107666015625;0.0084694499999999998951505375544002163223922252655029296875;-0.72603399999999995717558931573876179754734039306640625;-4.7420600000000003859668140648864209651947021484375;0.069490200000000001967492835319717414677143096923828125;-0.332739999999999980229148377475212328135967254638671875;0.4584289999999999754010104879853315651416778564453125;-1.0340100000000000957101065068854950368404388427734375;-0.436593999999999982097875772524275816977024078369140625;0.08706809999999999549746831917218514718115329742431640625;-1.1747900000000000009237055564881302416324615478515625;0.29503800000000002246025587737676687538623809814453125;0.648179999999999978399500832892954349517822265625;0.59697699999999997988453515063156373798847198486328125;-2.17555999999999993832489053602330386638641357421875;-1.1105899999999999661071115042432211339473724365234375;-0.429719000000000017625012560529285110533237457275390625;0.241839999999999999413802242997917346656322479248046875;0.161131999999999997452704292300040833652019500732421875;0.10325099999999999555999607991907396353781223297119140625;0.1906210000000000126529897670479840599000453948974609375;-2.56280999999999981042719809920527040958404541015625;0.428493999999999986005860819204826839268207550048828125;0.1659190000000000109192654917933396063745021820068359375;-0.041315499999999998059774242165076429955661296844482421875;-3.21201999999999987522869560052640736103057861328125;0.0165723000000000016129764190964124281890690326690673828125;-1.449510000000000076170181273482739925384521484375;-0.212716999999999989423571378210908733308315277099609375;0.096362000000000003208100451956852339208126068115234375;-0.1836109999999999964348518233236973173916339874267578125;-0.55453399999999997138644403094076551496982574462890625;0.33988600000000002143707433788222260773181915283203125;0.366640000000000021440627051561023108661174774169921875;1.1872499999999999165112285481882281601428985595703125;-7.00659999999999971720399116748012602329254150390625;0.8648160000000000291464630208793096244335174560546875;-4.08664999999999967172925607883371412754058837890625;0.1906569999999999931450389567544334568083286285400390625;0.438983999999999985330845220232731662690639495849609375;-0.66478899999999996328625684327562339603900909423828125;-0.1143470000000000041939784978239913471043109893798828125;0.12170599999999999474287193379495874978601932525634765625]
      mask Display: e = 0.06;c1 = [120 150 230]/255;c2 = ([120 150 230]+0)/383;c3 = ([120 150 230]+128)/383;patch([0 1 1 0],[0 0 1 1],c1);patch([0 1 1 1-e 1-e 0+e],[0 0 1 1-e 0+e 0+e],c2);patch([0 0 1 1-e 0+e 0+e],[0 1 1 1-e 1-e 0+e],c3);plot([0 1 1 0 0],[0 0 1 1 0]);disp('b');
  netsum : Sum  Inputs=2  SaturateOnIntegerOverflow=on  InputSameDT=on  OutDataTypeStr=Inherit: Same as first input
      mask Display: e = 0.06;c1 = [120 150 230]/255;c2 = ([120 150 230]+0)/383;c3 = ([120 150 230]+128)/383;patch([0 1 1 0],[0 0 1 1],c1);patch([0 1 1 1-e 1-e 0+e],[0 0 1 1-e 0+e 0+e],c2);patch([0 0 1 1-e 0+e 0+e],[0 1 1 1-e 1-e 0+e],c3);plot([0 1 1 0 0],[0 0 1 1 0]);disp('+');
  tansig : neural/Transfer Functions/tansig
      settings: SourceProductName=Deep Learning Toolbox
  "a{6}" : Outport  InitialOutput=[0;0;0;0;0;0;0;0;0;0;0;0;0;0;0;0;0;0;0;0;0;0;0;0;0;0;0;0;0;0;0;0;0;0;0;0;0;0;0;0;0;0;0;0;0;0;0;0;0;0]
      mask Display: e = 0.06;c1 = [120 230 180]/255;c2 = ([120 230 180]+0)/(256+128);c3 = ([120 230 180]+128)/(256+128);patch([0 1 1 0],[0 0 1 1],c1);patch([0 1 1 1-e 1-e 0+e],[0 0 1 1-e 0+e 0+e],c2);patch([0 0 1 1-e 0+e 0+e],[0 1 1 1-e 1-e 0+e],c3);plot([0 1 1 0 0],[0 0 1 1 0]);
  wires:
  tansig/1 -> "a{6}"/1
  netsum/1 -> tansig/1
  "b{6}"/1 -> netsum/2
  "LW{6,5}"/1("lz{6,5}") -> netsum/1
  Delays 1/1("pd{6,5}") -> "LW{6,5}"/1("ad{6,5}")
  "a{5} "/1 -> Delays 1/1("p{6}")

== system AcasXuClosedLoop_6/AcasXu_1_1/Layer 7 ==
  "a{6} " : Inport  PortDimensions=50
      mask Display: e = 0.06;c1 = [120 230 180]/255;c2 = ([120 230 180]+0)/(256+128);c3 = ([120 230 180]+128)/(256+128);patch([0 1 1 0],[0 0 1 1],c1);patch([0 1 1 1-e 1-e 0+e],[0 0 1 1-e 0+e 0+e],c2);patch([0 0 1 1-e 0+e 0+e],[0 1 1 1-e 1-e 0+e],c3);plot([0 1 1 0 0],[0 0 1 1 0]);
  Delays 1 : Subsystem
      mask Display: e = 0.06;c1 = [120 150 230]/255;c2 = ([120 150 230]+0)/383;c3 = ([120 150 230]+128)/383;patch([0 1 1 0],[0 0 1 1],c1);patch([0 1 1 1-e 1-e 0+e],[0 0 1 1-e 0+e 0+e],c2);patch([0 0 1 1-e 0+e 0+e],[0 1 1 1-e 1-e 0+e],c3);plot([0 1 1 0 0],[0 0 1 1 0]);disp('0');
  "LW{7,6}" : Subsystem
      mask Display: e = 0.06;c1 = [120 150 230]/255;c2 = ([120 150 230]+0)/383;c3 = ([120 150 230]+128)/383;patch([0 1 1 0],[0 0 1 1],c1);patch([0 1 1 1-e 1-e 0+e],[0 0 1 1-e 0+e 0+e],c2);patch([0 0 1 1-e 0+e 0+e],[0 1 1 1-e 1-e 0+e],c3);plot([0 1 1 0 0],[0 0 1 1 0]);disp('W');
  "b{7}" : Constant  Value=[-0.01028150000000000070798922280346232582814991474151611328125;-0.01586680000000000034798830483850906603038311004638671875;-0.01548229999999999918769422180275796563364565372467041015625;-0.01533600000000000067312821983023241045884788036346435546875;-0.0148281000000000003080646848729884368367493152618408203125]
      mask Display: e = 0.06;c1 = [120 150 230]/255;c2 = ([120 150 230]+0)/383;c3 = ([120 150 230]+128)/383;patch([0 1 1 0],[0 0 1 1],c1);patch([0 1 1 1-e 1-e 0+e],[0 0 1 1-e 0+e 0+e],c2);patch([0 0 1 1-e 0+e 0+e],[0 1 1 1-e 1-e 0+e],c3);plot([0 1 1 0 0],[0 0 1 1 0]);disp('b');
  netsum : Sum  Inputs=2  SaturateOnIntegerOverflow=on  InputSameDT=on  OutDataTypeStr=Inherit: Same as first input
      mask Display: e = 0.06;c1 = [120 150 230]/255;c2 = ([120 150 230]+0)/383;c3 = ([120 150 230]+128)/383;patch([0 1 1 0],[0 0 1 1],c1);patch([0 1 1 1-e 1-e 0+e],[0 0 1 1-e 0+e 0+e],c2);patch([0 0 1 1-e 0+e 0+e],[0 1 1 1-e 1-e 0+e],c3);plot([0 1 1 0 0],[0 0 1 1 0]);disp('+');
  purelin : neural/Transfer Functions/purelin
      settings: SourceProductName=Deep Learning Toolbox
  "a{7}" : Outport  InitialOutput=[0;0;0;0;0]
      mask Display: e = 0.06;c1 = [120 230 180]/255;c2 = ([120 230 180]+0)/(256+128);c3 = ([120 230 180]+128)/(256+128);patch([0 1 1 0],[0 0 1 1],c1);patch([0 1 1 1-e 1-e 0+e],[0 0 1 1-e 0+e 0+e],c2);patch([0 0 1 1-e 0+e 0+e],[0 1 1 1-e 1-e 0+e],c3);plot([0 1 1 0 0],[0 0 1 1 0]);
  wires:
  purelin/1 -> "a{7}"/1
  netsum/1 -> purelin/1
  "b{7}"/1 -> netsum/2
  "LW{7,6}"/1("lz{7,6}") -> netsum/1
  Delays 1/1("pd{7,6}") -> "LW{7,6}"/1("ad{7,6}")
  "a{6} "/1 -> Delays 1/1("p{7}")

== system AcasXuClosedLoop_6/AcasXu_1_1/Process Input 1 ==
  x : Inport  PortDimensions=5
      mask Display: e = 0.06;c1 = [120 230 180]/255;c2 = ([120 230 180]+0)/(256+128);c3 = ([120 230 180]+128)/(256+128);patch([0 1 1 0],[0 0 1 1],c1);patch([0 1 1 1-e 1-e 0+e],[0 0 1 1-e 0+e 0+e],c2);patch([0 0 1 1-e 0+e 0+e],[0 1 1 1-e 1-e 0+e],c3);plot([0 1 1 0 0],[0 0 1 1 0]);
  p : Outport  PortDimensions=5
      mask Display: e = 0.06;c1 = [120 230 180]/255;c2 = ([120 230 180]+0)/(256+128);c3 = ([120 230 180]+128)/(256+128);patch([0 1 1 0],[0 0 1 1],c1);patch([0 1 1 1-e 1-e 0+e],[0 0 1 1-e 0+e 0+e],c2);patch([0 0 1 1-e 0+e 0+e],[0 1 1 1-e 1-e 0+e],c3);plot([0 1 1 0 0],[0 0 1 1 0]);
  wires:
  x/1 -> p/1

== system AcasXuClosedLoop_6/AcasXu_1_1/Process Output 1 ==
  a : Inport  PortDimensions=5
      mask Display: e = 0.06;c1 = [120 230 180]/255;c2 = ([120 230 180]+0)/(256+128);c3 = ([120 230 180]+128)/(256+128);patch([0 1 1 0],[0 0 1 1],c1);patch([0 1 1 1-e 1-e 0+e],[0 0 1 1-e 0+e 0+e],c2);patch([0 0 1 1-e 0+e 0+e],[0 1 1 1-e 1-e 0+e],c3);plot([0 1 1 0 0],[0 0 1 1 0]);
  y : Outport  PortDimensions=5
      mask Display: e = 0.06;c1 = [120 230 180]/255;c2 = ([120 230 180]+0)/(256+128);c3 = ([120 230 180]+128)/(256+128);patch([0 1 1 0],[0 0 1 1],c1);patch([0 1 1 1-e 1-e 0+e],[0 0 1 1-e 0+e 0+e],c2);patch([0 0 1 1-e 0+e 0+e],[0 1 1 1-e 1-e 0+e],c3);plot([0 1 1 0 0],[0 0 1 1 0]);
  wires:
  a/1 -> y/1

== system AcasXuClosedLoop_6/networks/AcasXu_5_4 ==
  Input : Inport  PortDimensions=5
      mask Display: e = 0.06;c1 = [120 230 180]/255;c2 = ([120 230 180]+0)/(256+128);c3 = ([120 230 180]+128)/(256+128);patch([0 1 1 0],[0 0 1 1],c1);patch([0 1 1 1-e 1-e 0+e],[0 0 1 1-e 0+e 0+e],c2);patch([0 0 1 1-e 0+e 0+e],[0 1 1 1-e 1-e 0+e],c3);plot([0 1 1 0 0],[0 0 1 1 0]);
  Layer 1 : Subsystem
      mask Display: e = 0.06;c1 = [120 150 230]/255;c2 = ([120 150 230]+0)/383;c3 = ([120 150 230]+128)/383;patch([0 1 1 0],[0 0 1 1],c1);patch([0 1 1 1-e 1-e 0+e],[0 0 1 1-e 0+e 0+e],c2);patch([0 0 1 1-e 0+e 0+e],[0 1 1 1-e 1-e 0+e],c3);plot([0 1 1 0 0],[0 0 1 1 0]);
  Layer 2 : Subsystem
      mask Display: e = 0.06;c1 = [120 150 230]/255;c2 = ([120 150 230]+0)/383;c3 = ([120 150 230]+128)/383;patch([0 1 1 0],[0 0 1 1],c1);patch([0 1 1 1-e 1-e 0+e],[0 0 1 1-e 0+e 0+e],c2);patch([0 0 1 1-e 0+e 0+e],[0 1 1 1-e 1-e 0+e],c3);plot([0 1 1 0 0],[0 0 1 1 0]);
  Layer 3 : Subsystem
      mask Display: e = 0.06;c1 = [120 150 230]/255;c2 = ([120 150 230]+0)/383;c3 = ([120 150 230]+128)/383;patch([0 1 1 0],[0 0 1 1],c1);patch([0 1 1 1-e 1-e 0+e],[0 0 1 1-e 0+e 0+e],c2);patch([0 0 1 1-e 0+e 0+e],[0 1 1 1-e 1-e 0+e],c3);plot([0 1 1 0 0],[0 0 1 1 0]);
  Layer 4 : Subsystem
      mask Display: e = 0.06;c1 = [120 150 230]/255;c2 = ([120 150 230]+0)/383;c3 = ([120 150 230]+128)/383;patch([0 1 1 0],[0 0 1 1],c1);patch([0 1 1 1-e 1-e 0+e],[0 0 1 1-e 0+e 0+e],c2);patch([0 0 1 1-e 0+e 0+e],[0 1 1 1-e 1-e 0+e],c3);plot([0 1 1 0 0],[0 0 1 1 0]);
  Layer 5 : Subsystem
      mask Display: e = 0.06;c1 = [120 150 230]/255;c2 = ([120 150 230]+0)/383;c3 = ([120 150 230]+128)/383;patch([0 1 1 0],[0 0 1 1],c1);patch([0 1 1 1-e 1-e 0+e],[0 0 1 1-e 0+e 0+e],c2);patch([0 0 1 1-e 0+e 0+e],[0 1 1 1-e 1-e 0+e],c3);plot([0 1 1 0 0],[0 0 1 1 0]);
  Layer 6 : Subsystem
      mask Display: e = 0.06;c1 = [120 150 230]/255;c2 = ([120 150 230]+0)/383;c3 = ([120 150 230]+128)/383;patch([0 1 1 0],[0 0 1 1],c1);patch([0 1 1 1-e 1-e 0+e],[0 0 1 1-e 0+e 0+e],c2);patch([0 0 1 1-e 0+e 0+e],[0 1 1 1-e 1-e 0+e],c3);plot([0 1 1 0 0],[0 0 1 1 0]);
  Layer 7 : Subsystem
      mask Display: e = 0.06;c1 = [120 150 230]/255;c2 = ([120 150 230]+0)/383;c3 = ([120 150 230]+128)/383;patch([0 1 1 0],[0 0 1 1],c1);patch([0 1 1 1-e 1-e 0+e],[0 0 1 1-e 0+e 0+e],c2);patch([0 0 1 1-e 0+e 0+e],[0 1 1 1-e 1-e 0+e],c3);plot([0 1 1 0 0],[0 0 1 1 0]);
  Process Input 1 : Subsystem
      mask Display: e = 0.06;c1 = [120 150 230]/255;c2 = ([120 150 230]+0)/383;c3 = ([120 150 230]+128)/383;patch([0 1 1 0],[0 0 1 1],c1);patch([0 1 1 1-e 1-e 0+e],[0 0 1 1-e 0+e 0+e],c2);patch([0 0 1 1-e 0+e 0+e],[0 1 1 1-e 1-e 0+e],c3);plot([0 1 1 0 0],[0 0 1 1 0]);
  Process Output 1 : Subsystem
      mask Display: e = 0.06;c1 = [120 150 230]/255;c2 = ([120 150 230]+0)/383;c3 = ([120 150 230]+128)/383;patch([0 1 1 0],[0 0 1 1],c1);patch([0 1 1 1-e 1-e 0+e],[0 0 1 1-e 0+e 0+e],c2);patch([0 0 1 1-e 0+e 0+e],[0 1 1 1-e 1-e 0+e],c3);plot([0 1 1 0 0],[0 0 1 1 0]);
  Output : Outport  InitialOutput=[0;0;0;0;0]
      mask Display: e = 0.06;c1 = [120 230 180]/255;c2 = ([120 230 180]+0)/(256+128);c3 = ([120 230 180]+128)/(256+128);patch([0 1 1 0],[0 0 1 1],c1);patch([0 1 1 1-e 1-e 0+e],[0 0 1 1-e 0+e 0+e],c2);patch([0 0 1 1-e 0+e 0+e],[0 1 1 1-e 1-e 0+e],c3);plot([0 1 1 0 0],[0 0 1 1 0]);
  wires:
  Layer 7/1("a{7}") -> Process Output 1/1(a)
  [feedback6] -> Layer 7/1("a{6} ")
  Layer 6/1("a{6}") -> [feedback6]
  [feedback5] -> Layer 6/1("a{5} ")
  Layer 5/1("a{5}") -> [feedback5]
  [feedback4] -> Layer 5/1("a{4} ")
  Layer 4/1("a{4}") -> [feedback4]
  [feedback3] -> Layer 4/1("a{3} ")
  Layer 3/1("a{3}") -> [feedback3]
  [feedback2] -> Layer 3/1("a{2} ")
  Layer 2/1("a{2}") -> [feedback2]
  [feedback1] -> Layer 2/1("a{1} ")
  Layer 1/1("a{1}") -> [feedback1]
  Process Input 1/1(p) -> Layer 1/1("p{1}")
  Process Output 1/1(y) -> Output/1
  Input/1 -> Process Input 1/1(x)

== system AcasXuClosedLoop_6/AcasXu_1_1/Layer 1/Delays 1 ==
  "p{1}" : Inport  PortDimensions=5
      mask Display: e = 0.06;c1 = [120 230 180]/255;c2 = ([120 230 180]+0)/(256+128);c3 = ([120 230 180]+128)/(256+128);patch([0 1 1 0],[0 0 1 1],c1);patch([0 1 1 1-e 1-e 0+e],[0 0 1 1-e 0+e 0+e],c2);patch([0 0 1 1-e 0+e 0+e],[0 1 1 1-e 1-e 0+e],c3);plot([0 1 1 0 0],[0 0 1 1 0]);
  mux : Mux  Inputs=1
      mask Display: e = 0.06;c1 = [120 150 230]/255;c2 = ([120 150 230]+0)/383;c3 = ([120 150 230]+128)/383;patch([0 1 1 0],[0 0 1 1],c1);patch([0 1 1 1-e 1-e 0+e],[0 0 1 1-e 0+e 0+e],c2);patch([0 0 1 1-e 0+e 0+e],[0 1 1 1-e 1-e 0+e],c3);plot([0 1 1 0 0],[0 0 1 1 0]);disp('Mux')
  "pd{1,1}" : Outport
      mask Display: e = 0.06;c1 = [120 230 180]/255;c2 = ([120 230 180]+0)/(256+128);c3 = ([120 230 180]+128)/(256+128);patch([0 1 1 0],[0 0 1 1],c1);patch([0 1 1 1-e 1-e 0+e],[0 0 1 1-e 0+e 0+e],c2);patch([0 0 1 1-e 0+e 0+e],[0 1 1 1-e 1-e 0+e],c3);plot([0 1 1 0 0],[0 0 1 1 0]);
  wires:
  mux/1 -> "pd{1,1}"/1
  "p{1}"/1 -> mux/1
